simulink model "FaultCheck"  (R2022b)
settings: Solver=FixedStepAuto  StartTime=0.0  StopTime=10  FixedStep=1  RelTol=1e-3
undefined symbols (not defined in the file): C_Flt_IGBTULowerTempConfirmTh_u16, C_Flt_IGBTULowerTempDiagEn_b, C_Flt_IGBTULowerTempErrCode_u16, C_Flt_IGBTULowerTempPowerCoeff, C_Flt_IGBTULowerTempRecoveryTh_u16, C_Flt_IGBTULowerTempRecTh_s32, C_Flt_IGBTULowerTempTrigTh_s32, C_Flt_IGBTUOverTempConfirmTh_u16, C_Flt_IGBTUOverTempDiagEn_b, C_Flt_IGBTUOverTempErrCode_u16, C_Flt_IGBTUOverTempRecoveryTh_u16, C_Flt_IGBTUOverTempRecTh_s32, C_Flt_IGBTUOverTempTrigTh_s32, C_Flt_IGBTVLowerTempConfirmTh_u16, C_Flt_IGBTVLowerTempDiagEn_b, C_Flt_IGBTVLowerTempErrCode_u16, C_Flt_IGBTVLowerTempPowerCoeff, C_Flt_IGBTVLowerTempRecoveryTh_u16, C_Flt_IGBTVLowerTempRecTh_s32, C_Flt_IGBTVLowerTempTrigTh_s32, C_Flt_IGBTVOverTempConfirmTh_u16, C_Flt_IGBTVOverTempDiagEn_b, C_Flt_IGBTVOverTempErrCode_u16, C_Flt_IGBTVOverTempRecoveryTh_u16, C_Flt_IGBTVOverTempRecTh_s32, C_Flt_IGBTVOverTempTrigTh_s32, C_Flt_IGBTWLowerTempConfirmTh_u16, C_Flt_IGBTWLowerTempDiagEn_b, C_Flt_IGBTWLowerTempErrCode_u16, C_Flt_IGBTWLowerTempPowerCoeff, C_Flt_IGBTWLowerTempRecoveryTh_u16, C_Flt_IGBTWLowerTempRecTh_s32, C_Flt_IGBTWLowerTempTrigTh_s32, C_Flt_IGBTWOverTempConfirmTh_u16, C_Flt_IGBTWOverTempDiagEn_b, C_Flt_IGBTWOverTempErrCode_u16, C_Flt_IGBTWOverTempRecoveryTh_u16, C_Flt_IGBTWOverTempRecTh_s32, C_Flt_IGBTWOverTempTrigTh_s32, C_Flt_IuOCConfirmTh_u16, C_Flt_IuOCDiagEn_b, C_Flt_IuOCErrCode_u16, C_Flt_IuOCNegLimit_s32, C_Flt_IuOCPosLimit_s32, C_Flt_IuOCRecoveryTh_u16, C_Flt_IuZeroDriftDiagEn_b, C_Flt_IuZeroDriftErrCode_u16, C_Flt_IvOCConfirmTh_u16, C_Flt_IvOCDiagEn_b, C_Flt_IvOCErrCode_u16, C_Flt_IvOCNegLimit_s32, C_Flt_IvOCPosLimit_s32, C_Flt_IvOCRecoveryTh_u16, C_Flt_IvZeroDriftDiagEn_b, C_Flt_IvZeroDriftErrCode_u16, C_Flt_IwOCConfirmTh_u16, C_Flt_IwOCDiagEn_b, C_Flt_IwOCErrCode_u16, C_Flt_IwOCNegLimit_s32, C_Flt_IwOCPosLimit_s32 ... (+196)
libraries: YS_UserDefined_Library x21, simulink x5
(part 10 of 11)

== system FaultCheck/FaultDiag_HighTask_100us/FltDetn/ResolveSensorDetn/Flt_ResolveSensorDetn/Power Reduction Coefficient/If Action Subsystem1 ==
  PowRecCoef : Inport
  Action Port : ActionPort
  PowRecCoefOut : Outport
  wires:
  PowRecCoef/1 -> PowRecCoefOut/1

== system FaultCheck/FaultDiag_HighTask_100us/FltDetn/ResolveSensorDetn/Flt_ResolveSensorDetn/Power Reduction Coefficient/If Action Subsystem2 ==
  Action Port : ActionPort
  Constant1 : Constant  Value=FLT_COEF_ZERO
  PowRecCoefOut : Outport
  wires:
  Constant1/1 -> PowRecCoefOut/1

== system FaultCheck/FaultDiag_HighTask_100us/FltDetn/UdcDetn/UdcOverLim1Detn/ErrCode1/If Action Subsystem ==
  Action Port : ActionPort
  Assignment : Assignment  IndexMode=Zero-based  DiagnosticForDimensions=Warning  IndexOptions=Index vector (port)  Indices=1  OutputSizes=1
  Constant : Constant  Value=FLT_ERRCODE_0  OutDataTypeStr=fixdt('uint16', 'DataTypeOverride', 'Off')
  Constant1 : Constant  Value=FLT_ERRBIT_10
  Data Store Read : DataStoreRead  DataStoreName=Flt_ErrCode  IndexOptions=Index vector (dialog)  Indices=1  OutputSizes=1
  Data Store Write : DataStoreWrite  DataStoreName=Flt_ErrCode  IndexOptions=Index vector (dialog)  Indices=1  OutputSizes=1
  wires:
  Assignment/1 -> Data Store Write/1
  Constant/1 -> Assignment/2
  Data Store Read/1 -> Assignment/1
  Constant1/1 -> Assignment/3

== system FaultCheck/FaultDiag_HighTask_100us/FltDetn/UdcDetn/UdcOverLim1Detn/ErrCode1/If Action Subsystem1 ==
  ErrCod : Inport
  Action Port : ActionPort
  Assignment : Assignment  IndexMode=Zero-based  DiagnosticForDimensions=Warning  IndexOptions=Index vector (port)  Indices=1  OutputSizes=1
  Constant : Constant  Value=FLT_ERRBIT_10
  Data Store Read : DataStoreRead  DataStoreName=Flt_ErrCode  IndexOptions=Index vector (dialog)  Indices=1  OutputSizes=1
  Data Store Write : DataStoreWrite  DataStoreName=Flt_ErrCode  IndexOptions=Index vector (dialog)  Indices=1  OutputSizes=1
  wires:
  Constant/1 -> Assignment/3
  ErrCod/1 -> Assignment/2
  Assignment/1 -> Data Store Write/1
  Data Store Read/1 -> Assignment/1

== system FaultCheck/FaultDiag_HighTask_100us/FltDetn/UdcDetn/UdcOverLim1Detn/ErrDetn/If Action Subsystem ==
  Action Port : ActionPort
  Constant : Constant  Value=FLT_NOERR
  Out1 : Outport
  wires:
  Constant/1 -> Out1/1

== system FaultCheck/FaultDiag_HighTask_100us/FltDetn/UdcDetn/UdcOverLim1Detn/ErrDetn/If Action Subsystem1 ==
  InputVal : Inport
  OverLim1 : Inport  Port=2
  RecLim1 : Inport  Port=3
  CntrFltLim : Inport  Port=4
  CntrRecLim : Inport  Port=5
  Action Port : ActionPort
  Chart : Stateflow chart  TreatAsAtomicUnit=on
  Relational Operator1 : RelationalOperator  OutDataTypeStr=boolean  RndMeth=Simplest  InputSameDT=off
  Relational Operator2 : RelationalOperator  Operator=<=  OutDataTypeStr=boolean  RndMeth=Simplest  InputSameDT=off
  Terminator : Terminator
  FltFlg : Outport
  wires:
  OverLim1/1 -> Relational Operator1/2
  RecLim1/1 -> Relational Operator2/2
  Relational Operator1/1 -> Chart/1(FltInput)
  Relational Operator2/1 -> Chart/2(RecInput)
  CntrFltLim/1 -> Chart/3(CntrFltLim)
  CntrRecLim/1 -> Chart/4(CntrRecLim)
  Chart/2(FltFlg) -> FltFlg/1
  Chart/1(FunSt) -> Terminator/1
  InputVal/1 -> [InputVal], Relational Operator1/1
  [InputVal] -> Relational Operator2/1

== system FaultCheck/FaultDiag_HighTask_100us/FltDetn/UdcDetn/UdcOverLim1Detn/FltLvl/If Action Subsystem ==
  Action Port : ActionPort
  Constant : Constant  Value=FLTLVL_ZERO
  ValOut : Outport
  wires:
  Constant/1 -> ValOut/1

== system FaultCheck/FaultDiag_HighTask_100us/FltDetn/UdcDetn/UdcOverLim1Detn/FltLvl/If Action Subsystem1 ==
  In : Inport
  Action Port : ActionPort
  ValOut : Outport
  wires:
  In/1 -> ValOut/1

== system FaultCheck/FaultDiag_HighTask_100us/FltDetn/UdcDetn/UdcOverLim1Detn/Power Reduction Coefficient/If Action Subsystem ==
  Action Port : ActionPort
  Constant1 : Constant  Value=FLT_COEF_ONE
  PowRecCoefOut : Outport
  wires:
  Constant1/1 -> PowRecCoefOut/1

== system FaultCheck/FaultDiag_HighTask_100us/FltDetn/UdcDetn/UdcOverLim1Detn/Power Reduction Coefficient/If Action Subsystem1 ==
  PowRecCoef : Inport
  Action Port : ActionPort
  PowRecCoefOut : Outport
  wires:
  PowRecCoef/1 -> PowRecCoefOut/1

== system FaultCheck/FaultDiag_HighTask_100us/FltDetn/UdcDetn/UdcOverLim1Detn/Power Reduction Coefficient/If Action Subsystem2 ==
  Action Port : ActionPort
  Constant1 : Constant  Value=FLT_COEF_ZERO
  PowRecCoefOut : Outport
  wires:
  Constant1/1 -> PowRecCoefOut/1

== system FaultCheck/FaultDiag_HighTask_100us/FltDetn/UdcDetn/UdcOverLim2Detn/ErrCode1/If Action Subsystem ==
  Action Port : ActionPort
  Assignment : Assignment  IndexMode=Zero-based  DiagnosticForDimensions=Warning  IndexOptions=Index vector (port)  Indices=1  OutputSizes=1
  Constant : Constant  Value=FLT_ERRCODE_0  OutDataTypeStr=fixdt('uint16', 'DataTypeOverride', 'Off')
  Constant1 : Constant  Value=FLT_ERRBIT_74
  Data Store Read : DataStoreRead  DataStoreName=Flt_ErrCode  IndexOptions=Index vector (dialog)  Indices=1  OutputSizes=1
  Data Store Write : DataStoreWrite  DataStoreName=Flt_ErrCode  IndexOptions=Index vector (dialog)  Indices=1  OutputSizes=1
  wires:
  Assignment/1 -> Data Store Write/1
  Constant/1 -> Assignment/2
  Data Store Read/1 -> Assignment/1
  Constant1/1 -> Assignment/3

== system FaultCheck/FaultDiag_HighTask_100us/FltDetn/UdcDetn/UdcOverLim2Detn/ErrCode1/If Action Subsystem1 ==
  ErrCod : Inport
  Action Port : ActionPort
  Assignment : Assignment  IndexMode=Zero-based  DiagnosticForDimensions=Warning  IndexOptions=Index vector (port)  Indices=1  OutputSizes=1
  Constant : Constant  Value=FLT_ERRBIT_74
  Data Store Read : DataStoreRead  DataStoreName=Flt_ErrCode  IndexOptions=Index vector (dialog)  Indices=1  OutputSizes=1
  Data Store Write : DataStoreWrite  DataStoreName=Flt_ErrCode  IndexOptions=Index vector (dialog)  Indices=1  OutputSizes=1
  wires:
  Constant/1 -> Assignment/3
  ErrCod/1 -> Assignment/2
  Assignment/1 -> Data Store Write/1
  Data Store Read/1 -> Assignment/1

== system FaultCheck/FaultDiag_HighTask_100us/FltDetn/UdcDetn/UdcOverLim2Detn/ErrDetn/If Action Subsystem ==
  Action Port : ActionPort
  Constant : Constant  Value=FLT_NOERR
  Out1 : Outport
  wires:
  Constant/1 -> Out1/1

== system FaultCheck/FaultDiag_HighTask_100us/FltDetn/UdcDetn/UdcOverLim2Detn/ErrDetn/If Action Subsystem1 ==
  InputVal : Inport
  ErrDeb : Inport  Port=2
  Action Port : ActionPort
  Constant3 : Constant  Value=FLT_ERR
  Debounce : Subsystem
  Delay1 : Delay  DelayLength=1
  Signal Conversion : SignalConversion  OverrideOpt=off
  Switch2 : Switch  Criteria=u2 > Threshold  SaturateOnIntegerOverflow=off  InputSameDT=off
  Out1 : Outport
  wires:
  Signal Conversion/1 -> Out1/1
  ErrDeb/1 -> Debounce/2(ErrDeb)
  InputVal/1 -> Debounce/1(ErrInput)
  Debounce/1(ErrFlg) -> Switch2/2
  Switch2/1 -> Delay1/1, Signal Conversion/1
  Constant3/1 -> Switch2/1
  Delay1/1 -> Switch2/3

== system FaultCheck/FaultDiag_HighTask_100us/FltDetn/UdcDetn/UdcOverLim2Detn/FltLvl/If Action Subsystem ==
  Action Port : ActionPort
  Constant : Constant  Value=FLTLVL_ZERO
  ValOut : Outport
  wires:
  Constant/1 -> ValOut/1

== system FaultCheck/FaultDiag_HighTask_100us/FltDetn/UdcDetn/UdcOverLim2Detn/FltLvl/If Action Subsystem1 ==
  In : Inport
  Action Port : ActionPort
  ValOut : Outport
  wires:
  In/1 -> ValOut/1

== system FaultCheck/FaultDiag_HighTask_100us/FltDetn/UdcDetn/UdcOverLim2Detn/Power Reduction Coefficient/If Action Subsystem ==
  Action Port : ActionPort
  Constant1 : Constant  Value=FLT_COEF_ONE
  PowRecCoefOut : Outport
  wires:
  Constant1/1 -> PowRecCoefOut/1

== system FaultCheck/FaultDiag_HighTask_100us/FltDetn/UdcDetn/UdcOverLim2Detn/Power Reduction Coefficient/If Action Subsystem1 ==
  PowRecCoef : Inport
  Action Port : ActionPort
  PowRecCoefOut : Outport
  wires:
  PowRecCoef/1 -> PowRecCoefOut/1

== system FaultCheck/FaultDiag_HighTask_100us/FltDetn/UdcDetn/UdcOverLim2Detn/Power Reduction Coefficient/If Action Subsystem2 ==
  Action Port : ActionPort
  Constant1 : Constant  Value=FLT_COEF_ZERO
  PowRecCoefOut : Outport
  wires:
  Constant1/1 -> PowRecCoefOut/1

== system FaultCheck/FaultDiag_HighTask_100us/FltDetn/UdcDetn/UdcUnderLim1Detn/ErrCode1/If Action Subsystem ==
  Action Port : ActionPort
  Assignment : Assignment  IndexMode=Zero-based  DiagnosticForDimensions=Warning  IndexOptions=Index vector (port)  Indices=1  OutputSizes=1
  Constant : Constant  Value=FLT_ERRCODE_0  OutDataTypeStr=fixdt('uint16', 'DataTypeOverride', 'Off')
  Constant1 : Constant  Value=FLT_ERRBIT_11
  Data Store Read : DataStoreRead  DataStoreName=Flt_ErrCode  IndexOptions=Index vector (dialog)  Indices=1  OutputSizes=1
  Data Store Write : DataStoreWrite  DataStoreName=Flt_ErrCode  IndexOptions=Index vector (dialog)  Indices=1  OutputSizes=1
  wires:
  Assignment/1 -> Data Store Write/1
  Constant/1 -> Assignment/2
  Data Store Read/1 -> Assignment/1
  Constant1/1 -> Assignment/3

== system FaultCheck/FaultDiag_HighTask_100us/FltDetn/UdcDetn/UdcUnderLim1Detn/ErrCode1/If Action Subsystem1 ==
  ErrCod : Inport
  Action Port : ActionPort
  Assignment : Assignment  IndexMode=Zero-based  DiagnosticForDimensions=Warning  IndexOptions=Index vector (port)  Indices=1  OutputSizes=1
  Constant : Constant  Value=FLT_ERRBIT_11
  Data Store Read : DataStoreRead  DataStoreName=Flt_ErrCode  IndexOptions=Index vector (dialog)  Indices=1  OutputSizes=1
  Data Store Write : DataStoreWrite  DataStoreName=Flt_ErrCode  IndexOptions=Index vector (dialog)  Indices=1  OutputSizes=1
  wires:
  Constant/1 -> Assignment/3
  ErrCod/1 -> Assignment/2
  Assignment/1 -> Data Store Write/1
  Data Store Read/1 -> Assignment/1

== system FaultCheck/FaultDiag_HighTask_100us/FltDetn/UdcDetn/UdcUnderLim1Detn/ErrDetn/If Action Subsystem ==
  Action Port : ActionPort
  Constant : Constant  Value=FLT_NOERR
  Out1 : Outport
  wires:
  Constant/1 -> Out1/1

== system FaultCheck/FaultDiag_HighTask_100us/FltDetn/UdcDetn/UdcUnderLim1Detn/ErrDetn/If Action Subsystem1 ==
  InputVal : Inport
  LoLim1 : Inport  Port=2
  RecLim1 : Inport  Port=3
  CntrFltLim : Inport  Port=4
  CntrRecLim : Inport  Port=5
  Action Port : ActionPort
  Chart : Stateflow chart  TreatAsAtomicUnit=on
  Relational Operator1 : RelationalOperator  Operator=<=  OutDataTypeStr=boolean  RndMeth=Simplest  InputSameDT=off
  Relational Operator2 : RelationalOperator  OutDataTypeStr=boolean  RndMeth=Simplest  InputSameDT=off
  Terminator : Terminator
  FltFlg : Outport
  wires:
  [InputVal] -> Relational Operator2/1
  InputVal/1 -> Relational Operator1/1, [InputVal]
  Chart/1(FunSt) -> Terminator/1
  Chart/2(FltFlg) -> FltFlg/1
  CntrRecLim/1 -> Chart/4(CntrRecLim)
  CntrFltLim/1 -> Chart/3(CntrFltLim)
  Relational Operator2/1 -> Chart/2(RecInput)
  Relational Operator1/1 -> Chart/1(FltInput)
  RecLim1/1 -> Relational Operator2/2
  LoLim1/1 -> Relational Operator1/2

== system FaultCheck/FaultDiag_HighTask_100us/FltDetn/UdcDetn/UdcUnderLim1Detn/FltLvl/If Action Subsystem ==
  Action Port : ActionPort
  Constant : Constant  Value=FLTLVL_ZERO
  ValOut : Outport
  wires:
  Constant/1 -> ValOut/1

== system FaultCheck/FaultDiag_HighTask_100us/FltDetn/UdcDetn/UdcUnderLim1Detn/FltLvl/If Action Subsystem1 ==
  In : Inport
  Action Port : ActionPort
  ValOut : Outport
  wires:
  In/1 -> ValOut/1

== system FaultCheck/FaultDiag_HighTask_100us/FltDetn/UdcDetn/UdcUnderLim1Detn/Power Reduction Coefficient/If Action Subsystem ==
  Action Port : ActionPort
  Constant1 : Constant  Value=FLT_COEF_ONE
  PowRecCoefOut : Outport
  wires:
  Constant1/1 -> PowRecCoefOut/1

== system FaultCheck/FaultDiag_HighTask_100us/FltDetn/UdcDetn/UdcUnderLim1Detn/Power Reduction Coefficient/If Action Subsystem1 ==
  PowRecCoef : Inport
  Action Port : ActionPort
  PowRecCoefOut : Outport
  wires:
  PowRecCoef/1 -> PowRecCoefOut/1

== system FaultCheck/FaultDiag_HighTask_100us/FltDetn/UdcDetn/UdcUnderLim1Detn/Power Reduction Coefficient/If Action Subsystem2 ==
  Action Port : ActionPort
  Constant1 : Constant  Value=FLT_COEF_ZERO
  PowRecCoefOut : Outport
  wires:
  Constant1/1 -> PowRecCoefOut/1

== system FaultCheck/FaultDiag_HighTask_100us/FltDetn/UdcDetn/UdcUnderLim2Detn2/ErrCode1/If Action Subsystem ==
  Action Port : ActionPort
  Assignment : Assignment  IndexMode=Zero-based  DiagnosticForDimensions=Warning  IndexOptions=Index vector (port)  Indices=1  OutputSizes=1
  Constant : Constant  Value=FLT_ERRCODE_0  OutDataTypeStr=fixdt('uint16', 'DataTypeOverride', 'Off')
  Constant1 : Constant  Value=FLT_ERRBIT_30
  Data Store Read : DataStoreRead  DataStoreName=Flt_ErrCode  IndexOptions=Index vector (dialog)  Indices=1  OutputSizes=1
  Data Store Write : DataStoreWrite  DataStoreName=Flt_ErrCode  IndexOptions=Index vector (dialog)  Indices=1  OutputSizes=1
  wires:
  Assignment/1 -> Data Store Write/1
  Constant/1 -> Assignment/2
  Data Store Read/1 -> Assignment/1
  Constant1/1 -> Assignment/3

== system FaultCheck/FaultDiag_HighTask_100us/FltDetn/UdcDetn/UdcUnderLim2Detn2/ErrCode1/If Action Subsystem1 ==
  ErrCod : Inport
  Action Port : ActionPort
  Assignment : Assignment  IndexMode=Zero-based  DiagnosticForDimensions=Warning  IndexOptions=Index vector (port)  Indices=1  OutputSizes=1
  Constant : Constant  Value=FLT_ERRBIT_30
  Data Store Read : DataStoreRead  DataStoreName=Flt_ErrCode  IndexOptions=Index vector (dialog)  Indices=1  OutputSizes=1
  Data Store Write : DataStoreWrite  DataStoreName=Flt_ErrCode  IndexOptions=Index vector (dialog)  Indices=1  OutputSizes=1
  wires:
  Constant/1 -> Assignment/3
  ErrCod/1 -> Assignment/2
  Assignment/1 -> Data Store Write/1
  Data Store Read/1 -> Assignment/1

== system FaultCheck/FaultDiag_HighTask_100us/FltDetn/UdcDetn/UdcUnderLim2Detn2/ErrDetn/If Action Subsystem ==
  Action Port : ActionPort
  Constant : Constant  Value=FLT_NOERR
  Out1 : Outport
  wires:
  Constant/1 -> Out1/1

== system FaultCheck/FaultDiag_HighTask_100us/FltDetn/UdcDetn/UdcUnderLim2Detn2/ErrDetn/If Action Subsystem1 ==
  InputVal : Inport
  LoLim2 : Inport  Port=2
  RecLim2 : Inport  Port=3
  CntrFltLim : Inport  Port=4
  CntrRecLim : Inport  Port=5
  Action Port : ActionPort
  Chart : Stateflow chart  TreatAsAtomicUnit=on
  Relational Operator1 : RelationalOperator  Operator=<=  OutDataTypeStr=boolean  RndMeth=Simplest  InputSameDT=off
  Relational Operator2 : RelationalOperator  OutDataTypeStr=boolean  RndMeth=Simplest  InputSameDT=off
  Terminator : Terminator
  FltFlg : Outport
  wires:
  LoLim2/1 -> Relational Operator1/2
  RecLim2/1 -> Relational Operator2/2
  Relational Operator1/1 -> Chart/1(FltInput)
  Relational Operator2/1 -> Chart/2(RecInput)
  CntrFltLim/1 -> Chart/3(CntrFltLim)
  CntrRecLim/1 -> Chart/4(CntrRecLim)
  Chart/2(FltFlg) -> FltFlg/1
  Chart/1(FunSt) -> Terminator/1
  InputVal/1 -> [InputVal], Relational Operator1/1
  [InputVal] -> Relational Operator2/1

== system FaultCheck/FaultDiag_HighTask_100us/FltDetn/UdcDetn/UdcUnderLim2Detn2/FltLvl/If Action Subsystem ==
  Action Port : ActionPort
  Constant : Constant  Value=FLTLVL_ZERO
  ValOut : Outport
  wires:
  Constant/1 -> ValOut/1

== system FaultCheck/FaultDiag_HighTask_100us/FltDetn/UdcDetn/UdcUnderLim2Detn2/FltLvl/If Action Subsystem1 ==
  In : Inport
  Action Port : ActionPort
  ValOut : Outport
  wires:
  In/1 -> ValOut/1

== system FaultCheck/FaultDiag_HighTask_100us/FltDetn/UdcDetn/UdcUnderLim2Detn2/Power Reduction Coefficient/If Action Subsystem ==
  Action Port : ActionPort
  Constant1 : Constant  Value=FLT_COEF_ONE
  PowRecCoefOut : Outport
  wires:
  Constant1/1 -> PowRecCoefOut/1

== system FaultCheck/FaultDiag_HighTask_100us/FltDetn/UdcDetn/UdcUnderLim2Detn2/Power Reduction Coefficient/If Action Subsystem1 ==
  PowRecCoef : Inport
  Action Port : ActionPort
  PowRecCoefOut : Outport
  wires:
  PowRecCoef/1 -> PowRecCoefOut/1

== system FaultCheck/FaultDiag_HighTask_100us/FltDetn/UdcDetn/UdcUnderLim2Detn2/Power Reduction Coefficient/If Action Subsystem2 ==
  Action Port : ActionPort
  Constant1 : Constant  Value=FLT_COEF_ZERO
  PowRecCoefOut : Outport
  wires:
  Constant1/1 -> PowRecCoefOut/1

== system FaultCheck/FaultDiag_HighTask_100us/FltDetn/UdcZeroDrfDetn/UdcZeroDrfDetn/ErrCode1/If Action Subsystem ==
  Action Port : ActionPort
  Assignment : Assignment  IndexMode=Zero-based  DiagnosticForDimensions=Warning  IndexOptions=Index vector (port)  Indices=1  OutputSizes=1
  Constant : Constant  Value=FLT_ERRCODE_0
  Constant1 : Constant  Value=FLT_ERRBIT_55
  Data Store Read : DataStoreRead  DataStoreName=Flt_ErrCode  IndexOptions=Index vector (dialog)  Indices=1  OutputSizes=1
  Data Store Write : DataStoreWrite  DataStoreName=Flt_ErrCode  IndexOptions=Index vector (dialog)  Indices=1  OutputSizes=1
  wires:
  Constant1/1 -> Assignment/3
  Data Store Read/1 -> Assignment/1
  Constant/1 -> Assignment/2
  Assignment/1 -> Data Store Write/1

== system FaultCheck/FaultDiag_HighTask_100us/FltDetn/UdcZeroDrfDetn/UdcZeroDrfDetn/ErrCode1/If Action Subsystem1 ==
  ErrCod : Inport
  Action Port : ActionPort
  Assignment : Assignment  IndexMode=Zero-based  DiagnosticForDimensions=Warning  IndexOptions=Index vector (port)  Indices=1  OutputSizes=1
  Constant : Constant  Value=FLT_ERRBIT_55
  Data Store Read : DataStoreRead  DataStoreName=Flt_ErrCode  IndexOptions=Index vector (dialog)  Indices=1  OutputSizes=1
  Data Store Write : DataStoreWrite  DataStoreName=Flt_ErrCode  IndexOptions=Index vector (dialog)  Indices=1  OutputSizes=1
  wires:
  Data Store Read/1 -> Assignment/1
  Assignment/1 -> Data Store Write/1
  ErrCod/1 -> Assignment/2
  Constant/1 -> Assignment/3

== system FaultCheck/FaultDiag_HighTask_100us/FltDetn/UdcZeroDrfDetn/UdcZeroDrfDetn/ErrDetn/If Action Subsystem ==
  Action Port : ActionPort
  Constant : Constant  Value=FLT_NOERR
  Out1 : Outport
  wires:
  Constant/1 -> Out1/1

== system FaultCheck/FaultDiag_HighTask_100us/FltDetn/UdcZeroDrfDetn/UdcZeroDrfDetn/ErrDetn/If Action Subsystem1 ==
  InputVal : Inport
  Action Port : ActionPort
  Constant3 : Constant  Value=FLT_ERR
  Delay1 : Delay  DelayLength=1
  Switch2 : Switch  Criteria=u2 > Threshold  SaturateOnIntegerOverflow=off  InputSameDT=off
  Out1 : Outport
  wires:
  Delay1/1 -> Switch2/3
  Constant3/1 -> Switch2/1
  Switch2/1 -> Out1/1, Delay1/1
  InputVal/1 -> Switch2/2

== system FaultCheck/FaultDiag_HighTask_100us/FltDetn/UdcZeroDrfDetn/UdcZeroDrfDetn/FltLvl/If Action Subsystem ==
  Action Port : ActionPort
  Constant : Constant  Value=FLTLVL_ZERO
  ValOut : Outport
  wires:
  Constant/1 -> ValOut/1

== system FaultCheck/FaultDiag_HighTask_100us/FltDetn/UdcZeroDrfDetn/UdcZeroDrfDetn/FltLvl/If Action Subsystem1 ==
  In : Inport
  Action Port : ActionPort
  ValOut : Outport
  wires:
  In/1 -> ValOut/1

== system FaultCheck/FaultDiag_HighTask_100us/FltDetn/UdcZeroDrfDetn/UdcZeroDrfDetn/Power Reduction Coefficient/If Action Subsystem ==
  Action Port : ActionPort
  Constant1 : Constant  Value=FLT_COEF_ONE
  PowRecCoefOut : Outport
  wires:
  Constant1/1 -> PowRecCoefOut/1

== system FaultCheck/FaultDiag_HighTask_100us/FltDetn/UdcZeroDrfDetn/UdcZeroDrfDetn/Power Reduction Coefficient/If Action Subsystem1 ==
  PowRecCoef : Inport
  Action Port : ActionPort
  PowRecCoefOut : Outport
  wires:
  PowRecCoef/1 -> PowRecCoefOut/1

== system FaultCheck/FaultDiag_HighTask_100us/FltDetn/UdcZeroDrfDetn/UdcZeroDrfDetn/Power Reduction Coefficient/If Action Subsystem2 ==
  Action Port : ActionPort
  Constant1 : Constant  Value=FLT_COEF_ZERO
  PowRecCoefOut : Outport
  wires:
  Constant1/1 -> PowRecCoefOut/1

== system FaultCheck/FaultDiag_HighTask_100us/FltDetn/VoltagSensorDetn/Flt_VoltagSensorDetn/ErrCode/If Action Subsystem ==
  Action Port : ActionPort
  Assignment : Assignment  IndexMode=Zero-based  DiagnosticForDimensions=Warning  IndexOptions=Index vector (port)  Indices=1  OutputSizes=1
  Constant : Constant  Value=FLT_ERRCODE_0  OutDataTypeStr=fixdt('uint16', 'DataTypeOverride', 'Off')
  Constant1 : Constant  Value=FLT_ERRBIT_53
  Data Store Read : DataStoreRead  DataStoreName=Flt_ErrCode  IndexOptions=Index vector (dialog)  Indices=1  OutputSizes=1
  Data Store Write : DataStoreWrite  DataStoreName=Flt_ErrCode  IndexOptions=Index vector (dialog)  Indices=1  OutputSizes=1
  wires:
  Assignment/1 -> Data Store Write/1
  Constant/1 -> Assignment/2
  Data Store Read/1 -> Assignment/1
  Constant1/1 -> Assignment/3

== system FaultCheck/FaultDiag_HighTask_100us/FltDetn/VoltagSensorDetn/Flt_VoltagSensorDetn/ErrCode/If Action Subsystem1 ==
  ErrCod : Inport
  Action Port : ActionPort
  Assignment : Assignment  IndexMode=Zero-based  DiagnosticForDimensions=Warning  IndexOptions=Index vector (port)  Indices=1  OutputSizes=1
  Constant : Constant  Value=FLT_ERRBIT_53
  Data Store Read : DataStoreRead  DataStoreName=Flt_ErrCode  IndexOptions=Index vector (dialog)  Indices=1  OutputSizes=1
  Data Store Write : DataStoreWrite  DataStoreName=Flt_ErrCode  IndexOptions=Index vector (dialog)  Indices=1  OutputSizes=1
  wires:
  Constant/1 -> Assignment/3
  ErrCod/1 -> Assignment/2
  Assignment/1 -> Data Store Write/1
  Data Store Read/1 -> Assignment/1

== system FaultCheck/FaultDiag_HighTask_100us/FltDetn/VoltagSensorDetn/Flt_VoltagSensorDetn/ErrDetn/If Action Subsystem ==
  Action Port : ActionPort
  Constant : Constant  Value=FLT_NOERR
  Out1 : Outport
  wires:
  Constant/1 -> Out1/1

== system FaultCheck/FaultDiag_HighTask_100us/FltDetn/VoltagSensorDetn/Flt_VoltagSensorDetn/ErrDetn/If Action Subsystem1 ==
  InputVal : Inport
  ErrDeb : Inport  Port=2
  Action Port : ActionPort
  Constant3 : Constant  Value=FLT_ERR
  Debounce1 : Subsystem
  Delay1 : Delay  DelayLength=1
  Signal Conversion : SignalConversion  OverrideOpt=off
  Switch2 : Switch  Criteria=u2 > Threshold  SaturateOnIntegerOverflow=off  InputSameDT=off
  Out1 : Outport
  wires:
  Signal Conversion/1 -> Out1/1
  Delay1/1 -> Switch2/3
  Constant3/1 -> Switch2/1
  Switch2/1 -> Signal Conversion/1, Delay1/1
  Debounce1/1(ErrFlg) -> Switch2/2
  InputVal/1 -> Debounce1/1(ErrInput)
  ErrDeb/1 -> Debounce1/2(ErrDeb)

== system FaultCheck/FaultDiag_HighTask_100us/FltDetn/VoltagSensorDetn/Flt_VoltagSensorDetn/FltLvl/If Action Subsystem ==
  Action Port : ActionPort
  Constant : Constant  Value=FLTLVL_ZERO
  ValOut : Outport
  wires:
  Constant/1 -> ValOut/1

== system FaultCheck/FaultDiag_HighTask_100us/FltDetn/VoltagSensorDetn/Flt_VoltagSensorDetn/FltLvl/If Action Subsystem1 ==
  In : Inport
  Action Port : ActionPort
  ValOut : Outport
  wires:
  In/1 -> ValOut/1

== system FaultCheck/FaultDiag_HighTask_100us/FltDetn/VoltagSensorDetn/Flt_VoltagSensorDetn/Power Reduction Coefficient/If Action Subsystem ==
  Action Port : ActionPort
  Constant1 : Constant  Value=FLT_COEF_ONE
  PowRecCoefOut : Outport
  wires:
  Constant1/1 -> PowRecCoefOut/1

== system FaultCheck/FaultDiag_HighTask_100us/FltDetn/VoltagSensorDetn/Flt_VoltagSensorDetn/Power Reduction Coefficient/If Action Subsystem1 ==
  PowRecCoef : Inport
  Action Port : ActionPort
  PowRecCoefOut : Outport
  wires:
  PowRecCoef/1 -> PowRecCoefOut/1

== system FaultCheck/FaultDiag_HighTask_100us/FltDetn/VoltagSensorDetn/Flt_VoltagSensorDetn/Power Reduction Coefficient/If Action Subsystem2 ==
  Action Port : ActionPort
  Constant1 : Constant  Value=FLT_COEF_ZERO
  PowRecCoefOut : Outport
  wires:
  Constant1/1 -> PowRecCoefOut/1

== system FaultCheck/FaultDiagnose/PhaseCurrDiag/Flt_IuOverCurrDiag/Diagnose/Enable/FlgDebounce ==
  ConfirmTh : Inport
  RecoveryTh : Inport  Port=2
  IuOCFltFlgUnDeb : Inport  Port=3
  DebounceUnRec1 : YS_UserDefined_Library/Fault/DebounceUnRec  SystemSampleTime=-1  VariantActivationTime=update diagram  Latency=0  AutoFrameSizeCalculation=off
      settings: SourceProductName=YS
  Signal Copy : SignalConversion  OverrideOpt=off
  FlgOut : Outport
  wires:
  ConfirmTh/1 -> DebounceUnRec1/1
  IuOCFltFlgUnDeb/1 -> DebounceUnRec1/3
  DebounceUnRec1/1 -> Signal Copy/1  "M_Flt_IuOCFltFlgDeb_b"
  Signal Copy/1 -> FlgOut/1
  RecoveryTh/1 -> DebounceUnRec1/2

== system FaultCheck/FaultDiagnose/PhaseCurrDiag/Flt_IvOverCurrDiag/Diagnose/Enable/FlgDebounce ==
  ConfirmTh : Inport
  RecoveryTh : Inport  Port=2
  IvOCFltFlgRaw : Inport  Port=3
  DebounceUnRec : YS_UserDefined_Library/Fault/DebounceUnRec  SystemSampleTime=-1  VariantActivationTime=update diagram  Latency=0  AutoFrameSizeCalculation=off
      settings: SourceProductName=YS
  Signal Copy : SignalConversion  OverrideOpt=off
  FlgOut : Outport
  wires:
  Signal Copy/1 -> FlgOut/1
  DebounceUnRec/1 -> Signal Copy/1  "M_Flt_IvOCFltFlgDeb_b"
  IvOCFltFlgRaw/1 -> DebounceUnRec/3
  ConfirmTh/1 -> DebounceUnRec/1
  RecoveryTh/1 -> DebounceUnRec/2

== system FaultCheck/FaultDiagnose/PhaseCurrDiag/Flt_IwOverCurrDiag/Diagnose/Enable/FlgDebounce ==
  ConfirmTh : Inport
  RecoveryTh : Inport  Port=2
  IwOCFltFlgRaw : Inport  Port=3
  DebounceUnRec : YS_UserDefined_Library/Fault/DebounceUnRec  SystemSampleTime=-1  VariantActivationTime=update diagram  Latency=0  AutoFrameSizeCalculation=off
      settings: SourceProductName=YS
  Signal Copy : SignalConversion  OverrideOpt=off
  FlgOut : Outport
  wires:
  ConfirmTh/1 -> DebounceUnRec/1
  IwOCFltFlgRaw/1 -> DebounceUnRec/3
  DebounceUnRec/1 -> Signal Copy/1  "M_Flt_IwOCFltFlgDeb_b"
  Signal Copy/1 -> FlgOut/1
  RecoveryTh/1 -> DebounceUnRec/2

== system FaultCheck/FaultDiag_HighTask_100us/FltDetn/CurrentSensorDetn/Flt_CurrentSensorDetn/ErrDetn/If Action Subsystem1/Debounce1 ==
  ErrInput : Inport
  ErrDeb : Inport  Port=2
  Constant : Constant  Value=FLT_ZERO
  Constant1 : Constant  Value=FLT_ONE
  Data Type Conversion : DataTypeConversion  OutDataTypeStr=int8  SaturateOnIntegerOverflow=off  RndMeth=Floor
  Data Type Conversion1 : DataTypeConversion  OutDataTypeStr=uint8  SaturateOnIntegerOverflow=off  RndMeth=Floor
  Delay : Delay  DelayLength=1
  Min : MinMax  Inputs=2  OutDataTypeStr=int8
  Relational Operator : RelationalOperator  Operator=~=  OutDataTypeStr=boolean  RndMeth=Simplest  InputSameDT=off
  Relational Operator1 : RelationalOperator  OutDataTypeStr=boolean  RndMeth=Simplest  InputSameDT=off
  Sum : Sum
  Switch : Switch  Criteria=u2 ~= 0  OutDataTypeStr=int8  SaturateOnIntegerOverflow=off  InputSameDT=off
  ErrFlg : Outport
  wires:
  Data Type Conversion1/1 -> Delay/1
  Data Type Conversion/1 -> Min/2, Relational Operator1/2
  ErrInput/1 -> Relational Operator/1
  Constant/1 -> Relational Operator/2
  Relational Operator/1 -> Switch/3, Switch/2
  Constant1/1 -> Sum/2
  Delay/1 -> Sum/1
  Sum/1 -> Switch/1
  Switch/1 -> Min/1
  ErrDeb/1 -> Data Type Conversion/1
  Min/1 -> Relational Operator1/1, Data Type Conversion1/1
  Relational Operator1/1 -> ErrFlg/1

== system FaultCheck/FaultDiag_HighTask_100us/FltDetn/DriveUdcDetn/DriveUdcDetn/ErrDetn/If Action Subsystem1/Debounce1 ==
  ErrInput : Inport
  ErrDeb : Inport  Port=2
  Constant : Constant  Value=FLT_ZERO
  Constant1 : Constant  Value=FLT_ONE
  Delay : Delay  DelayLength=1
  Min : MinMax  Inputs=2  OutDataTypeStr=uint8
  Relational Operator : RelationalOperator  Operator=~=  OutDataTypeStr=boolean  RndMeth=Simplest  InputSameDT=off
  Relational Operator1 : RelationalOperator  OutDataTypeStr=boolean  RndMeth=Simplest  InputSameDT=off
  Sum : Sum
  Switch : Switch  Criteria=u2 ~= 0  OutDataTypeStr=uint8  SaturateOnIntegerOverflow=off  InputSameDT=off
  ErrFlg : Outport
  wires:
  Relational Operator1/1 -> ErrFlg/1
  Switch/1 -> Min/1
  Sum/1 -> Switch/1
  Delay/1 -> Sum/1
  Constant1/1 -> Sum/2
  Relational Operator/1 -> Switch/2, Switch/3
  Constant/1 -> Relational Operator/2
  ErrInput/1 -> Relational Operator/1
  ErrDeb/1 -> Relational Operator1/2, Min/2
  Min/1 -> Delay/1, Relational Operator1/1

== system FaultCheck/FaultDiag_HighTask_100us/FltDetn/Drive_H_Detn/Drive_H_Detn/ErrDetn/If Action Subsystem1/Debounce1 ==
  ErrInput : Inport
  ErrDeb : Inport  Port=2
  Constant : Constant  Value=FLT_ZERO
  Constant1 : Constant  Value=FLT_ONE
  Delay : Delay  DelayLength=1
  Min : MinMax  Inputs=2  OutDataTypeStr=uint8
  Relational Operator : RelationalOperator  Operator=~=  OutDataTypeStr=boolean  RndMeth=Simplest  InputSameDT=off
  Relational Operator1 : RelationalOperator  OutDataTypeStr=boolean  RndMeth=Simplest  InputSameDT=off
  Sum : Sum
  Switch : Switch  Criteria=u2 ~= 0  OutDataTypeStr=uint8  SaturateOnIntegerOverflow=off  InputSameDT=off
  ErrFlg : Outport
  wires:
  Relational Operator1/1 -> ErrFlg/1
  Switch/1 -> Min/1
  Sum/1 -> Switch/1
  Delay/1 -> Sum/1
  Constant1/1 -> Sum/2
  Relational Operator/1 -> Switch/2, Switch/3
  Constant/1 -> Relational Operator/2
  ErrInput/1 -> Relational Operator/1
  ErrDeb/1 -> Relational Operator1/2, Min/2
  Min/1 -> Delay/1, Relational Operator1/1

== system FaultCheck/FaultDiag_HighTask_100us/FltDetn/Drive_L_Detn/Drive_L_Detn/ErrDetn/If Action Subsystem1/Debounce1 ==
  ErrInput : Inport
  ErrDeb : Inport  Port=2
  Constant : Constant  Value=FLT_ZERO
  Constant1 : Constant  Value=FLT_ONE
  Delay : Delay  DelayLength=1
  Min : MinMax  Inputs=2  OutDataTypeStr=uint8
  Relational Operator : RelationalOperator  Operator=~=  OutDataTypeStr=boolean  RndMeth=Simplest  InputSameDT=off
  Relational Operator1 : RelationalOperator  OutDataTypeStr=boolean  RndMeth=Simplest  InputSameDT=off
  Sum : Sum
  Switch : Switch  Criteria=u2 ~= 0  OutDataTypeStr=uint8  SaturateOnIntegerOverflow=off  InputSameDT=off
  ErrFlg : Outport
  wires:
  Relational Operator1/1 -> ErrFlg/1
  Switch/1 -> Min/1
  Sum/1 -> Switch/1
  Delay/1 -> Sum/1
  Constant1/1 -> Sum/2
  Relational Operator/1 -> Switch/2, Switch/3
  Constant/1 -> Relational Operator/2
  ErrInput/1 -> Relational Operator/1
  ErrDeb/1 -> Relational Operator1/2, Min/2
  Min/1 -> Delay/1, Relational Operator1/1

== system FaultCheck/FaultDiag_HighTask_100us/FltDetn/HWOverCurrDetn/HWOverCurrDetn/ErrDetn/If Action Subsystem1/Debounce1 ==
  ErrInput : Inport
  ErrDeb : Inport  Port=2
  Constant : Constant  Value=FLT_ZERO
  Constant1 : Constant  Value=FLT_ONE
  Delay : Delay  DelayLength=1
  Min : MinMax  Inputs=2  OutDataTypeStr=uint8
  Relational Operator : RelationalOperator  Operator=~=  OutDataTypeStr=boolean  RndMeth=Simplest  InputSameDT=off
  Relational Operator1 : RelationalOperator  OutDataTypeStr=boolean  RndMeth=Simplest  InputSameDT=off
  Sum : Sum
  Switch : Switch  Criteria=u2 ~= 0  OutDataTypeStr=uint8  SaturateOnIntegerOverflow=off  InputSameDT=off
  ErrFlg : Outport
  wires:
  Relational Operator1/1 -> ErrFlg/1
  Switch/1 -> Min/1
  Sum/1 -> Switch/1
  Delay/1 -> Sum/1
  Constant1/1 -> Sum/2
  Relational Operator/1 -> Switch/2, Switch/3
  Constant/1 -> Relational Operator/2
  ErrInput/1 -> Relational Operator/1
  ErrDeb/1 -> Relational Operator1/2, Min/2
  Min/1 -> Delay/1, Relational Operator1/1

== system FaultCheck/FaultDiag_HighTask_100us/FltDetn/HWOverUdcDetn/HWOverCurrDetn/ErrDetn/If Action Subsystem1/Debounce1 ==
  ErrInput : Inport
  ErrDeb : Inport  Port=2
  Constant : Constant  Value=FLT_ZERO
  Constant1 : Constant  Value=FLT_ONE
  Delay : Delay  DelayLength=1
  Min : MinMax  Inputs=2  OutDataTypeStr=uint8
  Relational Operator : RelationalOperator  Operator=~=  OutDataTypeStr=boolean  RndMeth=Simplest  InputSameDT=off
  Relational Operator1 : RelationalOperator  OutDataTypeStr=boolean  RndMeth=Simplest  InputSameDT=off
  Sum : Sum
  Switch : Switch  Criteria=u2 ~= 0  OutDataTypeStr=uint8  SaturateOnIntegerOverflow=off  InputSameDT=off
  ErrFlg : Outport
  wires:
  Relational Operator1/1 -> ErrFlg/1
  Switch/1 -> Min/1
  Sum/1 -> Switch/1
  Delay/1 -> Sum/1
  Constant1/1 -> Sum/2
  Relational Operator/1 -> Switch/2, Switch/3
  Constant/1 -> Relational Operator/2
  ErrInput/1 -> Relational Operator/1
  ErrDeb/1 -> Relational Operator1/2, Min/2
  Min/1 -> Delay/1, Relational Operator1/1

== system FaultCheck/FaultDiag_HighTask_100us/FltDetn/OverCurrDetn/Flt_IuOverCurrDetn/ErrDetn1/If Action Subsystem1/Debounce1 ==
  ErrInput : Inport
  ErrDeb : Inport  Port=2
  Constant : Constant  Value=FLT_ZERO
  Constant1 : Constant  Value=FLT_ONE
  Delay : Delay  DelayLength=1
  Min : MinMax  Inputs=2  OutDataTypeStr=uint8
  Relational Operator : RelationalOperator  Operator=~=  OutDataTypeStr=boolean  RndMeth=Simplest  InputSameDT=off
  Relational Operator1 : RelationalOperator  OutDataTypeStr=boolean  RndMeth=Simplest  InputSameDT=off
  Sum : Sum
  Switch : Switch  Criteria=u2 ~= 0  OutDataTypeStr=uint8  SaturateOnIntegerOverflow=off  InputSameDT=off
  ErrFlg : Outport
  wires:
  Relational Operator1/1 -> ErrFlg/1
  Switch/1 -> Min/1
  Sum/1 -> Switch/1
  Delay/1 -> Sum/1
  Constant1/1 -> Sum/2
  Relational Operator/1 -> Switch/2, Switch/3
  Constant/1 -> Relational Operator/2
  ErrInput/1 -> Relational Operator/1
  ErrDeb/1 -> Relational Operator1/2, Min/2
  Min/1 -> Delay/1, Relational Operator1/1

== system FaultCheck/FaultDiag_HighTask_100us/FltDetn/OverCurrDetn/Flt_IvOverCurrDetn/ErrDetn1/If Action Subsystem1/Debounce1 ==
  ErrInput : Inport
  ErrDeb : Inport  Port=2
  Constant : Constant  Value=FLT_ZERO
  Constant1 : Constant  Value=FLT_ONE
  Delay : Delay  DelayLength=1
  Min : MinMax  Inputs=2  OutDataTypeStr=uint8
  Relational Operator : RelationalOperator  Operator=~=  OutDataTypeStr=boolean  RndMeth=Simplest  InputSameDT=off
  Relational Operator1 : RelationalOperator  OutDataTypeStr=boolean  RndMeth=Simplest  InputSameDT=off
  Sum : Sum
  Switch : Switch  Criteria=u2 ~= 0  OutDataTypeStr=uint8  SaturateOnIntegerOverflow=off  InputSameDT=off
  ErrFlg : Outport
  wires:
  Relational Operator1/1 -> ErrFlg/1
  Switch/1 -> Min/1
  Sum/1 -> Switch/1
  Delay/1 -> Sum/1
  Constant1/1 -> Sum/2
  Relational Operator/1 -> Switch/2, Switch/3
  Constant/1 -> Relational Operator/2
  ErrInput/1 -> Relational Operator/1
  ErrDeb/1 -> Relational Operator1/2, Min/2
  Min/1 -> Delay/1, Relational Operator1/1

== system FaultCheck/FaultDiag_HighTask_100us/FltDetn/OverCurrDetn/Flt_IwOverCurrDetn1/ErrDetn1/If Action Subsystem1/Debounce1 ==
  ErrInput : Inport
  ErrDeb : Inport  Port=2
  Constant : Constant  Value=FLT_ZERO
  Constant1 : Constant  Value=FLT_ONE
  Delay : Delay  DelayLength=1
  Min : MinMax  Inputs=2  OutDataTypeStr=uint8
  Relational Operator : RelationalOperator  Operator=~=  OutDataTypeStr=boolean  RndMeth=Simplest  InputSameDT=off
  Relational Operator1 : RelationalOperator  OutDataTypeStr=boolean  RndMeth=Simplest  InputSameDT=off
  Sum : Sum
  Switch : Switch  Criteria=u2 ~= 0  OutDataTypeStr=uint8  SaturateOnIntegerOverflow=off  InputSameDT=off
  ErrFlg : Outport
  wires:
  Relational Operator1/1 -> ErrFlg/1
  Switch/1 -> Min/1
  Sum/1 -> Switch/1
  Delay/1 -> Sum/1
  Constant1/1 -> Sum/2
  Relational Operator/1 -> Switch/2, Switch/3
  Constant/1 -> Relational Operator/2
  ErrInput/1 -> Relational Operator/1
  ErrDeb/1 -> Relational Operator1/2, Min/2
  Min/1 -> Delay/1, Relational Operator1/1

== system FaultCheck/FaultDiag_HighTask_100us/FltDetn/RecUDetn/RecUDetn/ErrDetn/If Action Subsystem1/Debounce ==
  ErrInput : Inport
  ErrDeb : Inport  Port=2
  Constant : Constant  Value=FLT_ZERO
  Constant1 : Constant  Value=FLT_ONE
  Delay : Delay  DelayLength=1
  Min : MinMax  Inputs=2  OutDataTypeStr=uint8
  Relational Operator : RelationalOperator  Operator=~=  OutDataTypeStr=boolean  RndMeth=Simplest  InputSameDT=off
  Relational Operator1 : RelationalOperator  OutDataTypeStr=boolean  RndMeth=Simplest  InputSameDT=off
  Sum : Sum
  Switch : Switch  Criteria=u2 ~= 0  OutDataTypeStr=uint8  SaturateOnIntegerOverflow=off  InputSameDT=off
  ErrFlg : Outport
  wires:
  Switch/1 -> Min/1
  Min/1 -> Delay/1, Relational Operator1/1
  ErrDeb/1 -> Min/2, Relational Operator1/2
  ErrInput/1 -> Relational Operator/1
  Constant/1 -> Relational Operator/2
  Relational Operator/1 -> Switch/3, Switch/2
  Constant1/1 -> Sum/2
  Delay/1 -> Sum/1
  Sum/1 -> Switch/1
  Relational Operator1/1 -> ErrFlg/1

== system FaultCheck/FaultDiag_HighTask_100us/FltDetn/ResolveSensorDetn/Flt_ResolveSensorDetn/ErrDetn/If Action Subsystem1/Debounce1 ==
  ErrInput : Inport
  ErrDeb : Inport  Port=2
  Constant : Constant  Value=FLT_ZERO
  Constant1 : Constant  Value=FLT_ONE
  Data Type Conversion : DataTypeConversion  OutDataTypeStr=int8  SaturateOnIntegerOverflow=off  RndMeth=Floor
  Data Type Conversion1 : DataTypeConversion  OutDataTypeStr=uint8  SaturateOnIntegerOverflow=off  RndMeth=Floor
  Delay : Delay  DelayLength=1
  Min : MinMax  Inputs=2  OutDataTypeStr=int8
  Relational Operator : RelationalOperator  Operator=~=  OutDataTypeStr=boolean  RndMeth=Simplest  InputSameDT=off
  Relational Operator1 : RelationalOperator  OutDataTypeStr=boolean  RndMeth=Simplest  InputSameDT=off
  Sum : Sum
  Switch : Switch  Criteria=u2 ~= 0  OutDataTypeStr=int8  SaturateOnIntegerOverflow=off  InputSameDT=off
  ErrFlg : Outport
  wires:
  Data Type Conversion1/1 -> Delay/1
  Data Type Conversion/1 -> Min/2, Relational Operator1/2
  ErrInput/1 -> Relational Operator/1
  Constant/1 -> Relational Operator/2
  Relational Operator/1 -> Switch/3, Switch/2
  Constant1/1 -> Sum/2
  Delay/1 -> Sum/1
  Sum/1 -> Switch/1
  Switch/1 -> Min/1
  ErrDeb/1 -> Data Type Conversion/1
  Min/1 -> Relational Operator1/1, Data Type Conversion1/1
  Relational Operator1/1 -> ErrFlg/1

== system FaultCheck/FaultDiag_HighTask_100us/FltDetn/UdcDetn/UdcOverLim2Detn/ErrDetn/If Action Subsystem1/Debounce ==
  ErrInput : Inport
  ErrDeb : Inport  Port=2
  Constant : Constant  Value=FLT_ZERO
  Constant1 : Constant  Value=FLT_ONE
  Delay : Delay  DelayLength=1
  Min : MinMax  Inputs=2  OutDataTypeStr=uint8
  Relational Operator : RelationalOperator  Operator=~=  OutDataTypeStr=boolean  RndMeth=Simplest  InputSameDT=off
  Relational Operator1 : RelationalOperator  OutDataTypeStr=boolean  RndMeth=Simplest  InputSameDT=off
  Sum : Sum
  Switch : Switch  Criteria=u2 ~= 0  OutDataTypeStr=uint8  SaturateOnIntegerOverflow=off  InputSameDT=off
  ErrFlg : Outport
  wires:
  Switch/1 -> Min/1
  Min/1 -> Delay/1, Relational Operator1/1
  ErrDeb/1 -> Min/2, Relational Operator1/2
  ErrInput/1 -> Relational Operator/1
  Constant/1 -> Relational Operator/2
  Relational Operator/1 -> Switch/3, Switch/2
  Constant1/1 -> Sum/2
  Delay/1 -> Sum/1
  Sum/1 -> Switch/1
  Relational Operator1/1 -> ErrFlg/1

== system FaultCheck/FaultDiag_HighTask_100us/FltDetn/VoltagSensorDetn/Flt_VoltagSensorDetn/ErrDetn/If Action Subsystem1/Debounce1 ==
  ErrInput : Inport
  ErrDeb : Inport  Port=2
  Constant : Constant  Value=FLT_ZERO
  Constant1 : Constant  Value=FLT_ONE
  Data Type Conversion : DataTypeConversion  OutDataTypeStr=int8  SaturateOnIntegerOverflow=off  RndMeth=Floor
  Data Type Conversion1 : DataTypeConversion  OutDataTypeStr=uint8  SaturateOnIntegerOverflow=off  RndMeth=Floor
  Delay : Delay  DelayLength=1
  Min : MinMax  Inputs=2  OutDataTypeStr=int8
  Relational Operator : RelationalOperator  Operator=~=  OutDataTypeStr=boolean  RndMeth=Simplest  InputSameDT=off
  Relational Operator1 : RelationalOperator  OutDataTypeStr=boolean  RndMeth=Simplest  InputSameDT=off
  Sum : Sum
  Switch : Switch  Criteria=u2 ~= 0  OutDataTypeStr=int8  SaturateOnIntegerOverflow=off  InputSameDT=off
  ErrFlg : Outport
  wires:
  Data Type Conversion1/1 -> Delay/1
  Data Type Conversion/1 -> Min/2, Relational Operator1/2
  ErrInput/1 -> Relational Operator/1
  Constant/1 -> Relational Operator/2
  Relational Operator/1 -> Switch/3, Switch/2
  Constant1/1 -> Sum/2
  Delay/1 -> Sum/1
  Sum/1 -> Switch/1
  Switch/1 -> Min/1
  ErrDeb/1 -> Data Type Conversion/1
  Min/1 -> Relational Operator1/1, Data Type Conversion1/1
  Relational Operator1/1 -> ErrFlg/1

== stateflow chart FaultCheck/FltCheck/Determination/Hysteresis/Hysteresis_Chart ==
  (default) -> (junction 7)
  (junction 7) -> (junction 9) [order 1] : [FastRecover_one == 1]
  (junction 7) -> (junction 15) [order 2]
  (junction 9) -> (junction 12) : {Out  = false}
  (junction 15) -> (junction 19) [order 1] : [Fail == true]
  (junction 15) -> (junction 40) [order 2] : {Clear = Clear + 1;
      | Set = 0;}
  (junction 19) -> (junction 21) : {Set = Set + 1;
      | Out = false;}
  (junction 40) -> (junction 44) [order 1] : [Clear > ClearTh]
  (junction 21) -> (junction 26) [order 1] : [Set > ConfirmTh]
  (junction 40) -> (junction 48) [order 2]
  (junction 44) -> (junction 46) : {Out = false}
  (junction 21) -> (junction 30) [order 2] : {Out = false;
      | Clear = 0;}
  (junction 26) -> (junction 28) : {Out = true}
  (junction 46) -> (junction 48)
  (junction 48) -> (junction 34)
  (junction 30) -> (junction 34)
  (junction 28) -> (junction 30)
  (junction 34) -> (junction 11)
  (junction 12) -> (junction 11)
  (junction 11) -> (junction 42)
  data: Fail input; ClearTh input; ConfirmTh input; FastRecover_one input; Out output =false; Set local =0; Clear local =0

== stateflow chart FaultCheck/OverDelay/Hysteresis/Hysteresis_Chart ==
  (default) -> (junction 7)
  (junction 7) -> (junction 9) [order 1] : [FastRecover_one == 1]
  (junction 7) -> (junction 15) [order 2]
  (junction 9) -> (junction 12) : {Out  = false}
  (junction 15) -> (junction 19) [order 1] : [Fail == true]
  (junction 15) -> (junction 40) [order 2] : {Clear = Clear + 1;
      | Set = 0;}
  (junction 19) -> (junction 21) : {Set = Set + 1;
      | Out = false;}
  (junction 40) -> (junction 44) [order 1] : [Clear > ClearTh]
  (junction 21) -> (junction 26) [order 1] : [Set > ConfirmTh]
  (junction 40) -> (junction 48) [order 2]
  (junction 44) -> (junction 46) : {Out = false}
  (junction 21) -> (junction 30) [order 2] : {Out = false;
      | Clear = 0;}
  (junction 26) -> (junction 28) : {Out = true}
  (junction 46) -> (junction 48)
  (junction 48) -> (junction 34)
  (junction 30) -> (junction 34)
  (junction 28) -> (junction 30)
  (junction 34) -> (junction 11)
  (junction 12) -> (junction 11)
  (junction 11) -> (junction 42)
  data: Fail input; ClearTh input; ConfirmTh input; FastRecover_one input; Out output =false; Set local =0; Clear local =0

== stateflow chart FaultCheck/LowerDelay/Hysteresis/Hysteresis_Chart ==
  (default) -> (junction 7)
  (junction 7) -> (junction 9) [order 1] : [FastRecover_one == 1]
  (junction 7) -> (junction 15) [order 2]
  (junction 9) -> (junction 12) : {Out  = false}
  (junction 15) -> (junction 19) [order 1] : [Fail == true]
  (junction 15) -> (junction 40) [order 2] : {Clear = Clear + 1;
      | Set = 0;}
  (junction 19) -> (junction 21) : {Set = Set + 1;
      | Out = false;}
  (junction 40) -> (junction 44) [order 1] : [Clear > ClearTh]
  (junction 21) -> (junction 26) [order 1] : [Set > ConfirmTh]
  (junction 40) -> (junction 48) [order 2]
  (junction 44) -> (junction 46) : {Out = false}
  (junction 21) -> (junction 30) [order 2] : {Out = false;
      | Clear = 0;}
  (junction 26) -> (junction 28) : {Out = true}
  (junction 46) -> (junction 48)
  (junction 48) -> (junction 34)
  (junction 30) -> (junction 34)
  (junction 28) -> (junction 30)
  (junction 34) -> (junction 11)
  (junction 12) -> (junction 11)
  (junction 11) -> (junction 42)
  data: Fail input; ClearTh input; ConfirmTh input; FastRecover_one input; Out output =false; Set local =0; Clear local =0

== stateflow chart FaultCheck/LowerDelay/Relay/Relay_Chart ==
  (default) -> (junction 41)
  (junction 41) -> (junction 43) [order 1] : [FltSrc <= FltTh]
  (junction 41) -> (junction 49) [order 2]
  (junction 43) -> (junction 45) : {Fail = 1}
  (junction 49) -> (junction 51) [order 1] : [FltSrc >= RecoverFltTh]
  (junction 49) -> (junction 56) [order 2]
  (junction 51) -> (junction 53) : {Fail = 0}
  (junction 56) -> (junction 58) [order 1] : [Faildelay == 1]
  (junction 56) -> (junction 47) [order 2] : {Fail = 0}
  (junction 58) -> (junction 60) : {Fail = 1}
  (junction 60) -> (junction 47)
  (junction 53) -> (junction 60)
  (junction 45) -> (junction 53)
  data: RecoverFltTh input; FltSrc input; FltTh input; Fail output; Faildelay input

== stateflow chart FaultCheck/FaultDiagnose/CurrZeroDriftFltDiag/IuZeroDriftDiag/Diagnose/Normal/Chart ==
  (default) -> (junction 3)
  (junction 3) -> (junction 5) [order 1] : [FltFlg == true]
  (junction 3) -> (junction 9) [order 2] : [FlgOut ==false]
  (junction 5) -> (junction 7) : {FlgOut = true}
  (junction 9) -> (junction 11)
  (junction 7) -> (junction 11)
  (junction 11) -> (junction 14)
  data: FltFlg input; FlgOut output =false

== stateflow chart FaultCheck/FaultDiag_HighTask_100us/FltDetn/UdcDetn/UdcOverLim1Detn/ErrDetn/If Action Subsystem1/Chart ==
  state Init
    en:
    FunSt=1;
    FltFlg=FLT_OFF;
    CntrErr=0;
    CntrRec=0;
  state DebounceFlt
    en:
    FunSt=2;
    FltFlg=FLT_OFF;
    CntrErr = CntrErr + 1;
    du:
    CntrErr = CntrErr + 1;
  state DebounceRec
    en:
    FunSt=4;
    FltFlg=FLT_ON;
    CntrRec = CntrRec + 1
    du:
    CntrRec = CntrRec + 1;
  state FltDetn
    en:
    FunSt=3;
    FltFlg=FLT_ON;
  (default) -> Init
  Init -> DebounceFlt : [FltInput==FLT_ON]
  DebounceFlt -> Init [order 2] : [FltInput==FLT_OFF]
  DebounceRec -> Init [order 1] : [CntrRec>=CntrRecLim]
  DebounceFlt -> FltDetn [order 1] : [CntrErr>=CntrFltLim]
  DebounceRec -> FltDetn [order 2] : [RecInput==FLT_OFF]
  FltDetn -> DebounceRec : [RecInput==FLT_ON]
  data: FltInput input; FunSt output; FltFlg output; CntrErr local; CntrRec local; RecInput input; CntrFltLim input; CntrRecLim input; FLT_ON constant uint8 =1; FLT_OFF constant uint8 =0

== stateflow chart FaultCheck/FaultDiag_HighTask_100us/FltDetn/UdcDetn/UdcUnderLim1Detn/ErrDetn/If Action Subsystem1/Chart ==
  state Init
    en:
    FunSt=1;
    FltFlg=FLT_OFF;
    CntrErr=0;
    CntrRec=0;
  state DebounceFlt
    en:
    FunSt=2;
    FltFlg=FLT_OFF;
    CntrErr = CntrErr + 1;
    du:
    CntrErr = CntrErr + 1;
  state DebounceRec
    en:
    FunSt=4;
    FltFlg=FLT_ON;
    CntrRec = CntrRec + 1
    du:
    CntrRec = CntrRec + 1;
  state FltDetn
    en:
    FunSt=3;
    FltFlg=FLT_ON;
  (default) -> Init
  Init -> DebounceFlt : [FltInput==FLT_ON]
  DebounceFlt -> Init [order 2] : [FltInput==FLT_OFF]
  DebounceRec -> Init [order 1] : [CntrRec>=CntrRecLim]
  DebounceFlt -> FltDetn [order 1] : [CntrErr>=CntrFltLim]
  DebounceRec -> FltDetn [order 2] : [RecInput==FLT_OFF]
  FltDetn -> DebounceRec : [RecInput==FLT_ON]
  data: FltInput input; FunSt output; FltFlg output; CntrErr local; CntrRec local; RecInput input; CntrFltLim input; CntrRecLim input; FLT_ON constant uint8 =1; FLT_OFF constant uint8 =0

== stateflow chart FaultCheck/FaultDiag_HighTask_100us/FltDetn/UdcDetn/UdcUnderLim2Detn2/ErrDetn/If Action Subsystem1/Chart ==
  state Init
    en:
    FunSt=1;
    FltFlg=FLT_OFF;
    CntrErr=0;
    CntrRec=0;
  state DebounceFlt
    en:
    FunSt=2;
    FltFlg=FLT_OFF;
    CntrErr = CntrErr + 1;
    du:
    CntrErr = CntrErr + 1;
  state DebounceRec
    en:
    FunSt=4;
    FltFlg=FLT_ON;
    CntrRec = CntrRec + 1
    du:
    CntrRec = CntrRec + 1;
  state FltDetn
    en:
    FunSt=3;
    FltFlg=FLT_ON;
  (default) -> Init
  Init -> DebounceFlt : [FltInput==FLT_ON]
  DebounceFlt -> Init [order 2] : [FltInput==FLT_OFF]
  DebounceRec -> Init [order 1] : [CntrRec>=CntrRecLim]
  DebounceFlt -> FltDetn [order 1] : [CntrErr>=CntrFltLim]
  DebounceRec -> FltDetn [order 2] : [RecInput==FLT_OFF]
  FltDetn -> DebounceRec : [RecInput==FLT_ON]
  data: FltInput input; FunSt output; FltFlg output; CntrErr local; CntrRec local; RecInput input; CntrFltLim input; CntrRecLim input; FLT_ON constant uint8 =1; FLT_OFF constant uint8 =0

== stateflow chart FaultCheck/FltCheck/Chart ==
  (default) -> (junction 3)
  (junction 3) -> (junction 6) [order 1] : [FastRecover_one == true]
  (junction 3) -> (junction 14) [order 2]
  (junction 6) -> (junction 8) : {FltFlag = false}
  (junction 14) -> (junction 16) [order 1] : [FltConfirmed == true]
  (junction 14) -> (junction 20) [order 2]
  (junction 16) -> (junction 18) : {FltFlag = true}
  (junction 18) -> (junction 20)
  (junction 20) -> (junction 5)
  (junction 8) -> (junction 5)
  data: FltConfirmed input; FastRecover_one input; FltFlag output
